simulink model "sendDataToXplane"  (R2022a)
settings: Solver=ode45  StartTime=0.0  StopTime=inf  FixedStep=2/100  RelTol=1e-3  EnableMultiTasking=on
libraries: etargetslib x1, simulink x1, sldrtlib x1, dspnetwork x1
settings Model: Creator=Flight Test Lab  LastModifiedBy=Ammar Abdurrauf
settings SolverCC: ConcurrentTasks=on  AlgebraicLoopSolver=TrustRegion  AutoInsertRateTranBlk=on  InsertRTBMode=Never (minimum delay)
settings DataIOCC: SaveFormat=StructureWithTime  ReturnWorkspaceOutputs=off
settings OptimizationCC: BlockReduction=off  DefaultUnderspecifiedDataType=single  OptimizeBlockIOStorage=off  BufferReuse=off  GlobalBufferReuse=off  ExpressionFolding=off  LocalBlockOutputs=off  LifeSpan=inf
settings DebuggingCC: UnconnectedInputMsg=warning  UnconnectedOutputMsg=warning  UnconnectedLineMsg=warning  SFExecutionAtInitializationDiag=none  SFMachineParentedDataDiag=warning  ArithmeticOperatorsInVariantConditions=warning
settings HardwareCC: ProdBitPerSizeT=32  ProdBitPerPtrDiffT=32  ProdWordSize=32  ProdHWDeviceType=Specified
settings SFSimCC: SimUseLocalCustomCode=off  CustomCodeUndefinedFunction=UseInterfaceOnly
settings RTWCC: Description=Generic Real-Time Target  RTWUseLocalCustomCode=off  RTWCompilerOptimization=on
settings CodeAppCC: MaxIdLength=95  StateflowObjectComments=on
settings GRTTargetCC: TargetLangStandard=C89/C90 (ANSI)

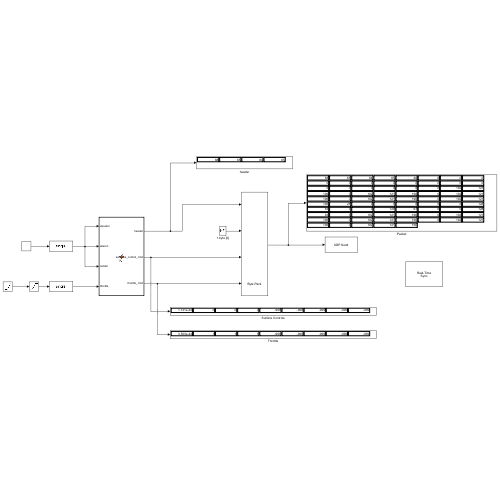
[thumbnail: Simulink's stored preview of the top-level diagram]
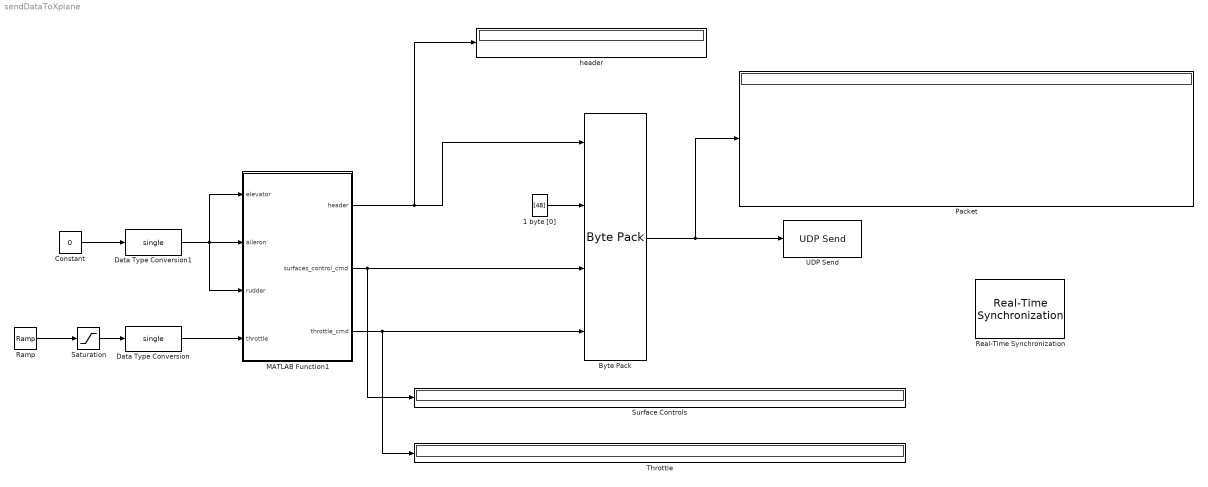
== system sendDataToXplane ==
  1 byte [0] : Constant  Value=[48]  OutDataTypeStr=uint8
  Byte Pack : etargetslib/Byte Pack  datatypes={'uint8','uint8','single','single'}  byteAlign=1
  Constant : Constant  Value=0
  Data Type Conversion : DataTypeConversion  OutDataTypeStr=single  SaturateOnIntegerOverflow=off  RndMeth=Floor
  Data Type Conversion1 : DataTypeConversion  OutDataTypeStr=single  SaturateOnIntegerOverflow=off  RndMeth=Floor
  MATLAB Function1 : MATLAB Function  TreatAsAtomicUnit=on
  Packet : Display
  Ramp : simulink/Sources/Ramp  slope=1  start=0  InitialOutput=0
  Real-Time Synchronization : sldrtlib/Real-Time Synchronization  SampleTime=0.00042  MaxMissedTicks=100  ShowMissedTicks=off  YieldWhenWaiting=off
  Saturation : Saturate  UpperLimit=1  LowerLimit=0
  Surface Controls : Display
  Throttle : Display
  UDP Send : dspnetwork/UDP Send  remoteURL='127.0.0.1'  remotePort=49000  localURL='0.0.0.0'  localPortSource=Automatically determine  localPort=-1  sendBufferSize=8192  sampletime=-1  blockPlatform=[]  separateLengthPort=0
  header : Display
  wires:
  Byte Pack/1 -> UDP Send/1, Packet/1
  MATLAB Function1/3(throttle_cmd) -> Throttle/1, Byte Pack/4
  1 byte [0]/1 -> Byte Pack/2
  MATLAB Function1/1(header) -> Byte Pack/1, header/1
  MATLAB Function1/2(surfaces_control_cmd) -> Surface Controls/1, Byte Pack/3
  Data Type Conversion/1 -> MATLAB Function1/4(throttle)
  Constant/1 -> Data Type Conversion1/1
  Data Type Conversion1/1 -> MATLAB Function1/3(rudder), MATLAB Function1/1(elevator), MATLAB Function1/2(aileron)
  Ramp/1 -> Saturation/1
  Saturation/1 -> Data Type Conversion/1

== matlab function sendDataToXplane/MATLAB Function1 ==
  data: elevator input; header output uint8; surfaces_control_cmd output; aileron input single; rudder input single; throttle input; throttle_cmd output single
function [header,surfaces_control_cmd,throttle_cmd] = fcn(elevator, aileron, rudder, throttle) 
header =[uint8(68) uint8(65) uint8(84) uint8(65)];
No_Comand = single(-999);
 %Surface_header = typecast(uint8([uint8(8) uint8(0) uint8(0) uint8(0)]),'single')
surfaces_control_cmd = [1.1210388e-44 elevator aileron rudder No_Comand No_Comand No_Comand No_Comand No_Comand  ];
%Throttle_header = typecast(uint8([uint8(25) uint8(0) uint8(0) uint8(0)]),'single');
throttle_cmd = [3.503246160812043e-44 throttle throttle throttle No_Comand No_Comand No_Comand No_Comand No_Comand];
end
